simulink model "ParachuteShcokLoadSimulation"  (R2022b)
settings: Solver=VariableStepAuto  StartTime=0.0  StopTime=10.0  RelTol=1e-3
values from neighbouring files (symbols this model uses):
  A_b = 0.01824    [Recovery_ShockLoad_Variables.m]
  Cdb = 0.54    [Recovery_ShockLoad_Variables.m]
  g = 9.81    [Recovery_ShockLoad_Variables.m]
  k = Es*A_sc/L    (= 11430)    [Recovery_ShockLoad_Variables.m]
  L = 12    [Recovery_ShockLoad_Variables.m]
  mb = 38    [Recovery_ShockLoad_Variables.m]
  mp = 1.47    [Recovery_ShockLoad_Variables.m]
  V_0 = 75    [Recovery_ShockLoad_Variables.m]
settings Model: Creator=mohka  LastModifiedBy=mohka

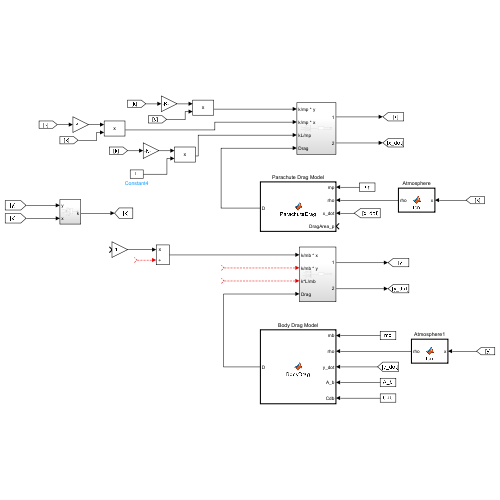
[thumbnail: Simulink's stored preview of the top-level diagram]
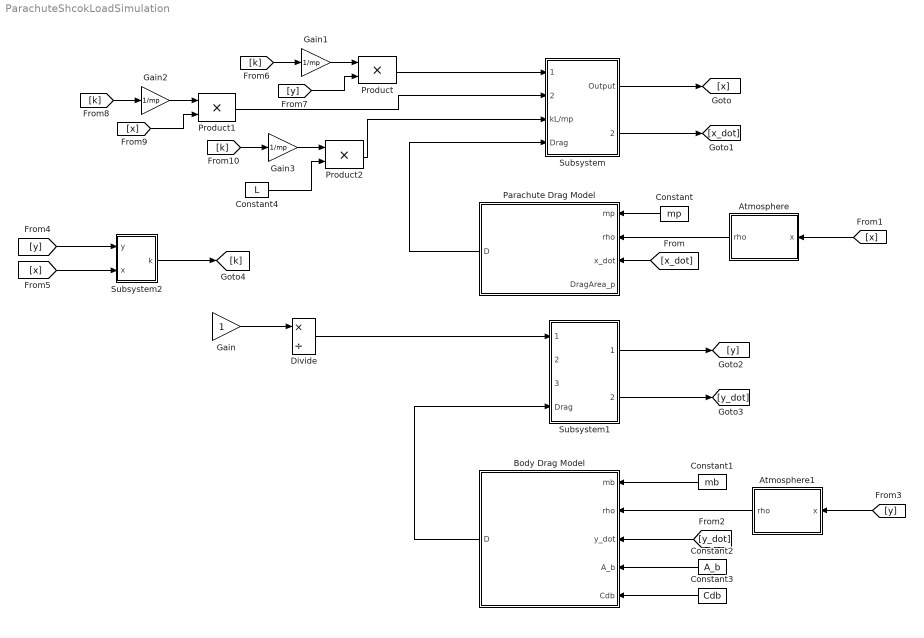
== system ParachuteShcokLoadSimulation ==
  Atmosphere : MATLAB Function  TreatAsAtomicUnit=on
  Atmosphere1 : MATLAB Function  TreatAsAtomicUnit=on
  Body Drag Model : MATLAB Function  TreatAsAtomicUnit=on
  Constant : Constant  Value=mp
  Constant1 : Constant  Value=mb
  Constant2 : Constant  Value=A_b
  Constant3 : Constant  Value=Cdb
  Constant4 : Constant  Value=L
  Divide : Product  Inputs=*/
  Gain : Gain
  Gain1 : Gain  Gain=1/mp
  Gain2 : Gain  Gain=1/mp
  Gain3 : Gain  Gain=1/mp
  Parachute Drag Model : MATLAB Function  TreatAsAtomicUnit=on
  Product : Product
  Product1 : Product
  Product2 : Product
  Subsystem : Subsystem
  Subsystem1 : Subsystem
  Subsystem2 : Subsystem
  wires:
  Product/1 -> Subsystem/1(k/mp * y)
  Product1/1 -> Subsystem/2(k/mp * x)
  Product2/1 -> Subsystem/3(kL/mp)
  Parachute Drag Model/1(D) -> Subsystem/4(Drag)
  Subsystem/1(Output) -> [x]
  Subsystem/2(Output1) -> [x_dot]
  [x_dot] -> Parachute Drag Model/3(x_dot)
  Constant/1 -> Parachute Drag Model/1(mp)
  [x] -> Atmosphere/1(x)
  Divide/1 -> Subsystem1/1(k/mb * x)
  ? -> Subsystem1/2(k/mb * y)
  ? -> Subsystem1/3(k*L/mb)
  Subsystem1/1(Output) -> [y]
  Subsystem1/2(Output1) -> [y_dot]
  Body Drag Model/1(D) -> Subsystem1/4(Drag)
  [y_dot] -> Body Drag Model/3(y_dot)
  Constant1/1 -> Body Drag Model/1(mb)
  Atmosphere/1(rho) -> Parachute Drag Model/2(rho)
  Atmosphere1/1(rho) -> Body Drag Model/2(rho)
  Constant2/1 -> Body Drag Model/4(A_b)
  Constant3/1 -> Body Drag Model/5(Cdb)
  [y] -> Atmosphere1/1(x)
  [y] -> Subsystem2/1(y)
  [x] -> Subsystem2/2(x)
  Subsystem2/1(k) -> [k]
  Gain/1 -> Divide/1
  ? -> Divide/2
  [k] -> Gain1/1
  Gain1/1 -> Product/1
  [y] -> Product/2
  [x] -> Product1/2
  [k] -> Gain2/1
  Gain2/1 -> Product1/1
  Constant4/1 -> Product2/2
  [k] -> Gain3/1
  Gain3/1 -> Product2/1

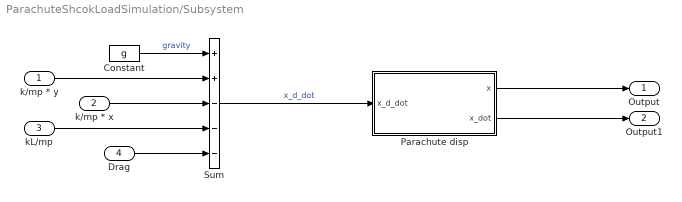
== system ParachuteShcokLoadSimulation/Subsystem ==
  k/mp * y : Inport
  k/mp * x : Inport  Port=2
  kL/mp : Inport  Port=3
  Drag : Inport  Port=4
  Constant : Constant  Value=g
  Parachute disp : Subsystem
  Sum : Sum  Inputs=++---
  Output : Outport
  Output1 : Outport  Port=2
  wires:
  Sum/1 -> Parachute disp/1(x_d_dot)  "x_d_dot"
  k/mp * y/1 -> Sum/2
  Drag/1 -> Sum/5
  k/mp * x/1 -> Sum/3
  kL/mp/1 -> Sum/4
  Parachute disp/1(x) -> Output/1
  Constant/1 -> Sum/1  "gravity"
  Parachute disp/2(x_dot) -> Output1/1

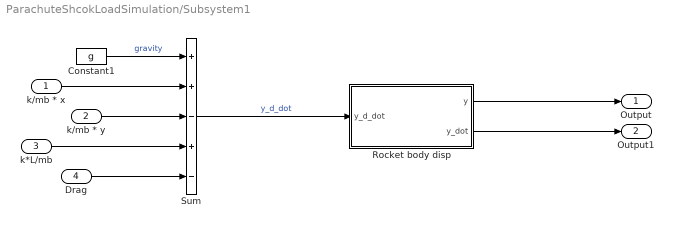
== system ParachuteShcokLoadSimulation/Subsystem1 ==
  k/mb * x : Inport
  k/mb * y : Inport  Port=2
  k*L/mb : Inport  Port=3
  Drag : Inport  Port=4
  Constant1 : Constant  Value=g
  Rocket body disp : Subsystem
  Sum : Sum  Inputs=++-+-
  Output : Outport
  Output1 : Outport  Port=2
  wires:
  k*L/mb/1 -> Sum/4
  Constant1/1 -> Sum/1  "gravity"
  k/mb * y/1 -> Sum/3
  Rocket body disp/1(y) -> Output/1
  k/mb * x/1 -> Sum/2
  Rocket body disp/2(y_dot) -> Output1/1
  Drag/1 -> Sum/5
  Sum/1 -> Rocket body disp/1(y_d_dot)  "y_d_dot"

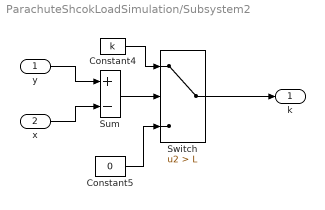
== system ParachuteShcokLoadSimulation/Subsystem2 ==
  y : Inport
  x : Inport  Port=2
  Constant4 : Constant  Value=k
  Constant5 : Constant  Value=0
  Sum : Sum  Inputs=+-
  Switch : Switch  Criteria=u2 > Threshold  Threshold=L  SaturateOnIntegerOverflow=off  InputSameDT=off
  k : Outport
  wires:
  Sum/1 -> Switch/2
  Switch/1 -> k/1
  Constant4/1 -> Switch/1
  Constant5/1 -> Switch/3
  x/1 -> Sum/2
  y/1 -> Sum/1

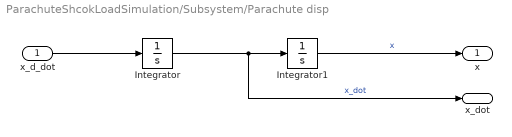
== system ParachuteShcokLoadSimulation/Subsystem/Parachute disp ==
  x_d_dot : Inport
  Integrator : Integrator  InitialCondition=V_0
  Integrator1 : Integrator
  x : Outport
  x_dot : Outport  Port=2
  wires:
  Integrator1/1 -> x/1  "x"
  x_d_dot/1 -> Integrator/1
  Integrator/1 -> x_dot/1, Integrator1/1  "x_dot"

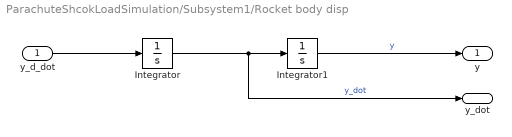
== system ParachuteShcokLoadSimulation/Subsystem1/Rocket body disp ==
  y_d_dot : Inport
  Integrator : Integrator  InitialCondition=V_0
  Integrator1 : Integrator
  y : Outport
  y_dot : Outport  Port=2
  wires:
  Integrator1/1 -> y/1  "y"
  y_d_dot/1 -> Integrator/1
  Integrator/1 -> y_dot/1, Integrator1/1  "y_dot"

== matlab function ParachuteShcokLoadSimulation/Atmosphere ==
  data: x input; rho output
function rho = fcn(x)

[~, ~, ~, rho] = atmosisa(3000-x);

== matlab function ParachuteShcokLoadSimulation/Parachute Drag Model ==
  data: mp input; D output; rho input; x_dot input; DragArea_p input
function D = ParachuteDrag(mp, rho, x_dot, DragArea_p)

D = 1/(2*mp) * rho * x_dot^2 * DragArea_p;

== matlab function ParachuteShcokLoadSimulation/Body Drag Model ==
  data: mb input; D output; rho input; y_dot input; A_b input; Cdb input
function D = BodyDrag(mb, rho, y_dot, A_b, Cdb)

D = 1/(2*mp) * rho * y_dot^2 * A_b * Cdb;

== matlab function ParachuteShcokLoadSimulation/Atmosphere1 ==
  data: x input; rho output
function rho = fcn(x)

[~, ~, ~, rho] = atmosisa(3000-x);
